simulink model "sEMG_DRL_LSTM"  (R2020a)
settings: Solver=VariableStepAuto  StartTime=0.0  StopTime=Tf  RelTol=1e-3
libraries: simulink x4, cstblocks x1, rllib x1
settings Model: Creator=DELL  LastModifiedBy=DELL

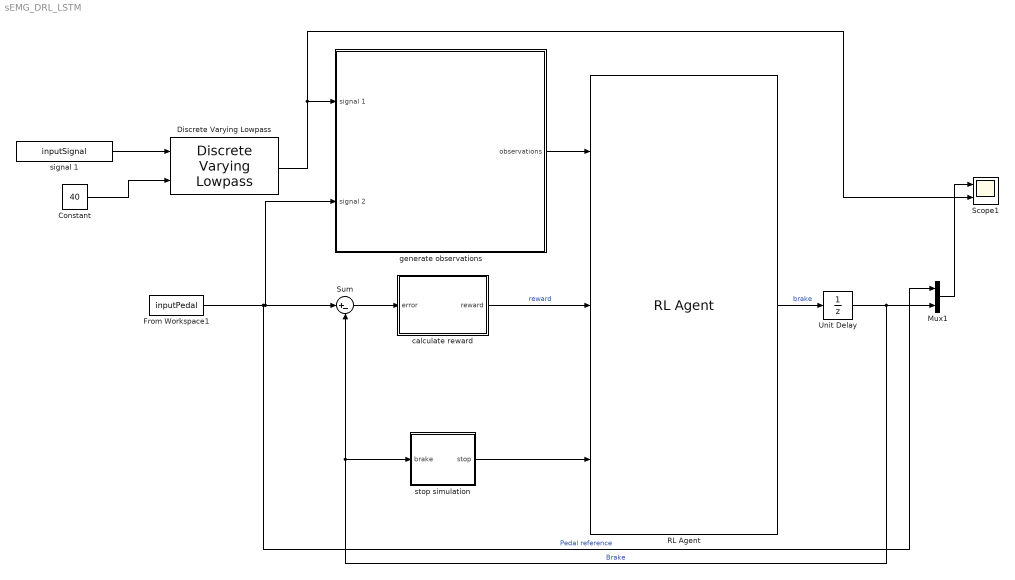
== system sEMG_DRL_LSTM ==
  Constant : Constant  Value=40
  Discrete Varying Lowpass : cstblocks/Linear Parameter Varying/Discrete Varying Lowpass  N=1  w0=0  Ts=1
      settings: SourceProductBaseCode=CT
  From Workspace1 : FromWorkspace  VariableName=inputPedal
  Mux1 : Mux  Inputs=2
  RL Agent : rllib/RL Agent  Agent=agent  ProvideReward=on  ProvideIsDone=on  ProvideCumRwd=off  TreatAsDirectFeedthrough=on  CollectLoggedSignals=on  CollectModelStates=on
  Scope1 : Scope  NumInputPorts=2
  Sum : Sum  Inputs=|+-
  Unit Delay : UnitDelay  SampleTime=0.01  HasFrameUpgradeWarning=on
  calculate reward : Subsystem
  generate observations : Subsystem
  signal 1 : FromWorkspace  VariableName=inputSignal
  stop simulation : Subsystem
  wires:
  Mux1/1 -> Scope1/1
  From Workspace1/1 -> Mux1/1, generate observations/2(signal 2), Sum/1  "Pedal reference"
  RL Agent/1 -> Unit Delay/1  "brake"
  calculate reward/1(reward) -> RL Agent/2  "reward"
  Sum/1 -> calculate reward/1(error)
  stop simulation/1(stop) -> RL Agent/3
  Unit Delay/1 -> Sum/2, stop simulation/1(brake), Mux1/2  "Brake"
  generate observations/1(observations) -> RL Agent/1
  signal 1/1 -> Discrete Varying Lowpass/1
  Discrete Varying Lowpass/1 -> Scope1/2, generate observations/1(signal 1)
  Constant/1 -> Discrete Varying Lowpass/2

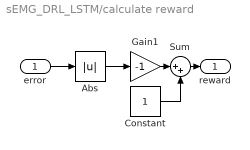
== system sEMG_DRL_LSTM/calculate reward ==
  error : Inport
  Abs : Abs
  Constant : Constant
  Gain1 : Gain  Gain=-1
  Sum : Sum  Inputs=|++
  reward : Outport  VectorParamsAs1DForOutWhenUnconnected=off
  wires:
  Abs/1 -> Gain1/1
  error/1 -> Abs/1
  Sum/1 -> reward/1
  Gain1/1 -> Sum/1
  Constant/1 -> Sum/2

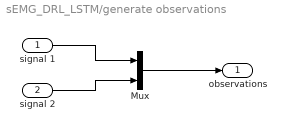
== system sEMG_DRL_LSTM/generate observations ==
  signal 1 : Inport
  signal 2 : Inport  Port=2
  Mux : Mux  Inputs=2
  observations : Outport  VectorParamsAs1DForOutWhenUnconnected=off
  wires:
  signal 1/1 -> Mux/1
  Mux/1 -> observations/1
  signal 2/1 -> Mux/2

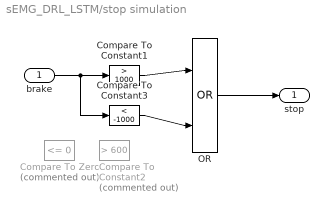
== system sEMG_DRL_LSTM/stop simulation ==
  brake : Inport
  Compare To Constant1 : simulink/Logic and Bit Operations/Compare To Constant  relop=>  const=1000  OutDataTypeStr=boolean
  Compare To Constant2 : simulink/Logic and Bit Operations/Compare To Constant  Commented=on  relop=>  const=600  OutDataTypeStr=boolean
  Compare To Constant3 : simulink/Logic and Bit Operations/Compare To Constant  relop=<  const=-1000  OutDataTypeStr=boolean
  Compare To Zero : simulink/Logic and Bit Operations/Compare To Zero  Commented=on  relop=<=  OutDataTypeStr=boolean
  OR : Logic  Operator=OR  IconShape=distinctive  AllPortsSameDT=off  OutDataTypeStr=boolean
  stop : Outport  VectorParamsAs1DForOutWhenUnconnected=off
  wires:
  brake/1 -> Compare To Constant3/1, Compare To Constant1/1
  Compare To Constant3/1 -> OR/2
  Compare To Constant1/1 -> OR/1
  OR/1 -> stop/1
